simulink model "openMHA_test_db_ar_gaintable"  (R2020b)
settings: Solver=VariableStepAuto  StartTime=0.0  StopTime=stop_time  RelTol=1e-3
InitFcn:
  | initCallback
StopFcn:
  | stopCallback
values from neighbouring files (symbols this model uses):
  buf_a = 65.*ones(num_bands,1)    [test_db_ar_gaintable_init.m]
  n_ar = num_bands*2    (= 16)    [test_db_ar_gaintable_init.m]
  num_bands = 8    [test_db_ar_gaintable_init.m]
  RAM_addresses = 2^(RAM_size)    (= 256)    [test_db_ar_gaintable_init.m]
  table_length = length(gtdata)    [test_db_ar_gaintable_init.m]
  X_high = 93    [test_db_ar_gaintable_init.m]
undefined symbols (not defined in the file or in its folder): xIn
libraries: dspsrcs4 x4, FPGA_Open_Speech_Tools x4, simulink x4, hdlsllib x2
settings Model: SimulationMode=accelerator  PacingRate=200  Creator=t96f346  LastModifiedBy=tyler

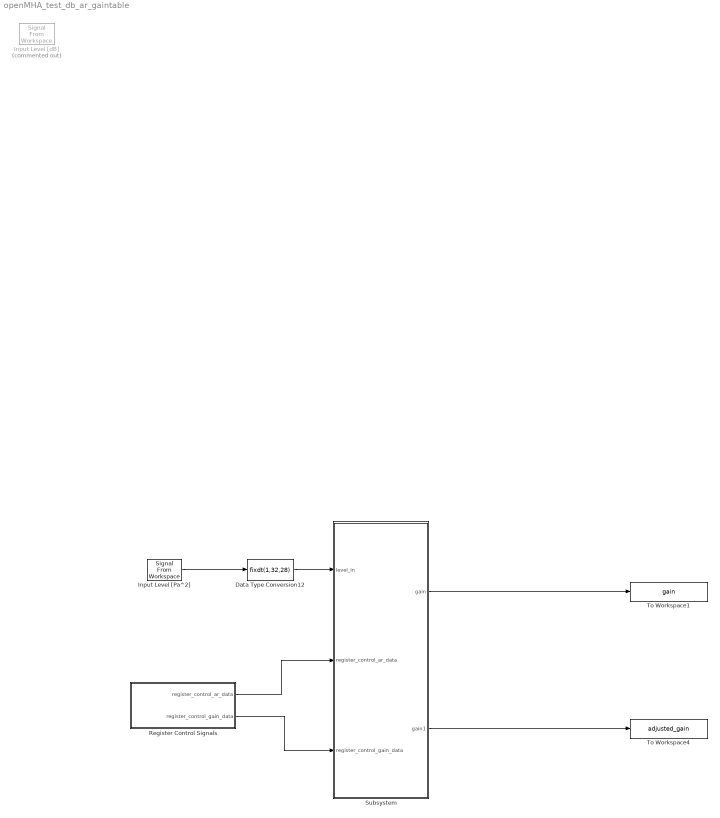
== system openMHA_test_db_ar_gaintable ==
  Data Type Conversion12 : DataTypeConversion  OutDataTypeStr=fixdt(1,32,28)
  Input Level [Pa^2] : dspsrcs4/Signal From Workspace  X=level_in  Ts=1  nsamps=1  OutputAfterFinalValue=Setting to zero  ignoreOrWarnInputAndFrameLengths=off  OutputFrames=off
  Input Level [dB] : dspsrcs4/Signal From Workspace  Commented=on  X=Lst  Ts=1  nsamps=1  OutputAfterFinalValue=Setting to zero  ignoreOrWarnInputAndFrameLengths=off  OutputFrames=off
  Register Control Signals : Subsystem
  Subsystem : Subsystem
  To Workspace1 : ToWorkspace  VariableName=gain  SampleTime=-1
      settings: Save2DSignal=2-D array (concatenate along first dimension)
  To Workspace4 : ToWorkspace  VariableName=adjusted_gain  SampleTime=-1
      settings: Save2DSignal=2-D array (concatenate along first dimension)
  wires:
  Input Level [Pa^2]/1 -> Data Type Conversion12/1
  Data Type Conversion12/1 -> Subsystem/1(level_in)
  Subsystem/1(gain) -> To Workspace1/1
  Subsystem/2(gain1) -> To Workspace4/1
  Register Control Signals/1("register_control_ar_data ") -> Subsystem/2(register_control_ar_data)
  Register Control Signals/2(register_control_gain_data) -> Subsystem/3(register_control_gain_data)

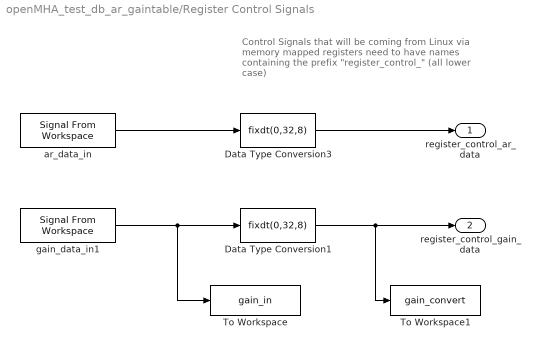
== system openMHA_test_db_ar_gaintable/Register Control Signals ==
  note: Control Signals that will be coming from Linux via
      | memory mapped registers need to have names
      | containing the prefix "register_control_"
      | (all lower case)
  Data Type Conversion1 : DataTypeConversion  OutDataTypeStr=fixdt(0,32,8)
  Data Type Conversion3 : DataTypeConversion  OutDataTypeStr=fixdt(0,32,8)
  To Workspace : ToWorkspace  VariableName=gain_in  SaveFormat=Timeseries  SampleTime=-1
  To Workspace1 : ToWorkspace  VariableName=gain_convert  SaveFormat=Timeseries  SampleTime=-1
  ar_data_in : dspsrcs4/Signal From Workspace  X=ar_data_in  Ts=1  nsamps=1  OutputAfterFinalValue=Setting to zero  ignoreOrWarnInputAndFrameLengths=off  OutputFrames=off
  gain_data_in1 : dspsrcs4/Signal From Workspace  X=gain_data_in  Ts=1  nsamps=1  OutputAfterFinalValue=Setting to zero  ignoreOrWarnInputAndFrameLengths=off  OutputFrames=off
  "register_control_ar_data " : Outport  VectorParamsAs1DForOutWhenUnconnected=off
  register_control_gain_data : Outport  Port=2  VectorParamsAs1DForOutWhenUnconnected=off
  wires:
  Data Type Conversion3/1 -> "register_control_ar_data "/1
  Data Type Conversion1/1 -> To Workspace1/1, register_control_gain_data/1
  ar_data_in/1 -> Data Type Conversion3/1
  gain_data_in1/1 -> To Workspace/1, Data Type Conversion1/1

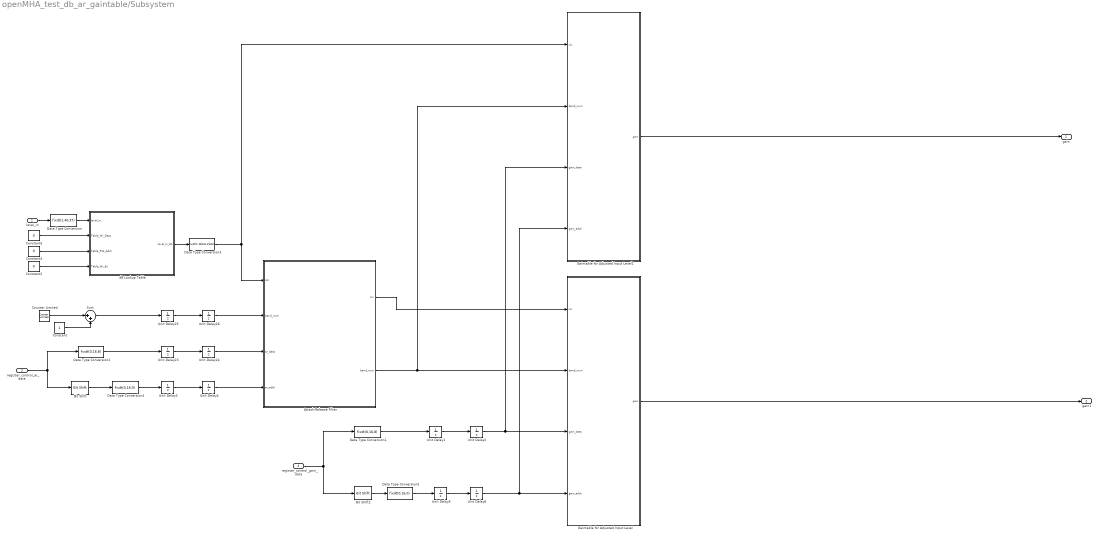
== system openMHA_test_db_ar_gaintable/Subsystem ==
  level_in : Inport
  register_control_ar_data : Inport  Port=2
  register_control_gain_data : Inport  Port=3
  Attack-Release Filter : Subsystem
  Bit Shift : hdlsllib/Logic and Bit Operations/Bit Shift  mode=Shift Right Logical  N=8
  Bit Shift1 : hdlsllib/Logic and Bit Operations/Bit Shift  mode=Shift Right Logical  N=8
  Constant : Constant
  Constant2 : Constant  Value=0  OutDataTypeStr=boolean  SampleTime=-1
  Constant4 : Constant  Value=0  OutDataTypeStr=uint16  SampleTime=-1
  Constant5 : Constant  Value=0  OutDataTypeStr=fixdt(1,40,32)  SampleTime=-1
  Counter Limited : simulink/Sources/Counter Limited  uplimit=num_bands-1  tsamp=-1
  Data Type Conversion : DataTypeConversion  OutDataTypeStr=fixdt(1,40,37)
  Data Type Conversion1 : DataTypeConversion  OutDataTypeStr=fixdt(0,16,8)
  Data Type Conversion2 : DataTypeConversion  OutDataTypeStr=fixdt(0,16,8)
  Data Type Conversion3 : DataTypeConversion  OutDataTypeStr=fixdt(1,Wbits,Fbits)
  Data Type Conversion4 : DataTypeConversion  OutDataTypeStr=fixdt(0,16,0)
  Data Type Conversion5 : DataTypeConversion  OutDataTypeStr=fixdt(0,16,0)
  Gaintable for Adjusted Input Level : Subsystem
  Gaintable for Adjusted Input Level1 : Subsystem
  Sum : Sum  Inputs=|++
  Unit Delay{1..6,23..26} (10 alike) : UnitDelay  SampleTime=-1  HasFrameUpgradeWarning=on
  dB Lookup Table : Subsystem
  gain : Outport
  gain1 : Outport  Port=2
  wires:
  Unit Delay24/1 -> Attack-Release Filter/3(ar_data)
  Data Type Conversion3/1 -> Attack-Release Filter/1(Lst), Gaintable for Adjusted Input Level1/1(Lin)
  Unit Delay26/1 -> Attack-Release Filter/2(band_num)
  Attack-Release Filter/1(Lin) -> Gaintable for Adjusted Input Level/1(Lin)
  Attack-Release Filter/2("band_num ") -> Gaintable for Adjusted Input Level1/2(band_num), Gaintable for Adjusted Input Level/2(band_num)
  Constant2/1 -> dB Lookup Table/4(Table_Wr_En)
  dB Lookup Table/1(level_in_db) -> Data Type Conversion3/1
  Data Type Conversion2/1 -> Unit Delay23/1
  Sum/1 -> Unit Delay25/1
  Unit Delay25/1 -> Unit Delay26/1
  Unit Delay23/1 -> Unit Delay24/1
  Gaintable for Adjusted Input Level1/1(gain) -> gain/1
  Constant5/1 -> dB Lookup Table/2(Table_Wr_Data)
  Gaintable for Adjusted Input Level/1(gain) -> gain1/1
  Constant4/1 -> dB Lookup Table/3(Table_RW_Addr)
  level_in/1 -> Data Type Conversion/1
  Data Type Conversion/1 -> dB Lookup Table/1(level_in)
  Counter Limited/1 -> Sum/1
  Constant/1 -> Sum/2
  register_control_ar_data/1 -> Data Type Conversion2/1, Bit Shift/1
  Unit Delay1/1 -> Unit Delay2/1
  Data Type Conversion1/1 -> Unit Delay1/1
  register_control_gain_data/1 -> Data Type Conversion1/1, Bit Shift1/1
  Unit Delay2/1 -> Gaintable for Adjusted Input Level1/3(gain_data), Gaintable for Adjusted Input Level/3(gain_data)
  Unit Delay3/1 -> Unit Delay4/1
  Unit Delay4/1 -> Attack-Release Filter/4(ar_addr)
  Unit Delay5/1 -> Unit Delay6/1
  Unit Delay6/1 -> Gaintable for Adjusted Input Level1/4(gain_addr), Gaintable for Adjusted Input Level/4(gain_addr)
  Bit Shift/1 -> Data Type Conversion4/1
  Data Type Conversion4/1 -> Unit Delay3/1
  Bit Shift1/1 -> Data Type Conversion5/1
  Data Type Conversion5/1 -> Unit Delay5/1

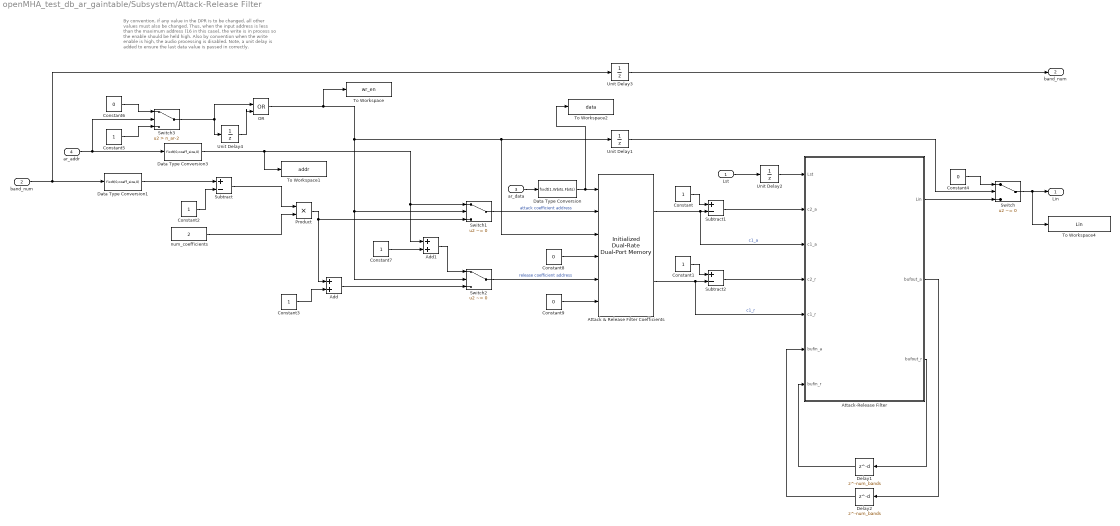
== system openMHA_test_db_ar_gaintable/Subsystem/Attack-Release Filter ==
  note: By convention, if any value in the DPR is to be changed, all other
      | values must also be changed.  Thus, when the input address is
      | less than the maximum address (16 in this case), the write is in
      | process so the enable should be held high.  Also by convention
      | when the write enable is high, the audio processing is disabled.
      | Note, a unit delay is added to ensure the last data value is passed
      | in correctly.
  Lst : Inport
  band_num : Inport  Port=2
  ar_data : Inport  Port=3
  ar_addr : Inport  Port=4
  Add : Sum
  Add1 : Sum
  Attack & Release Filter Coefficients : FPGA_Open_Speech_Tools/Initialized Dual-Rate Dual-Port Memory  ram_size=coeff_size  Table_Init=ar_coeffs
      settings: SourceProductName=FPGA Open Speech Tools
  Attack-Release Filter : Subsystem
  Constant : Constant  OutDataTypeStr=fixdt(1,Wbits,Fbits)  SampleTime=-1
  Constant1 : Constant  OutDataTypeStr=fixdt(1,Wbits,Fbits)  SampleTime=-1
  Constant2 : Constant  OutDataTypeStr=fixdt(0,coeff_size,0)  SampleTime=-1
  Constant3 : Constant  OutDataTypeStr=fixdt(0,coeff_size,0)  SampleTime=-1
  Constant4 : Constant  Value=0  OutDataTypeStr=fixdt(1,Wbits,Fbits)  SampleTime=-1
  Constant5 : Constant  OutDataTypeStr=boolean  SampleTime=-1
  Constant6 : Constant  Value=0  OutDataTypeStr=boolean  SampleTime=-1
  Constant7 : Constant  OutDataTypeStr=fixdt(0,coeff_size,0)  SampleTime=-1
  Constant8 : Constant  Value=0  OutDataTypeStr=fixdt(1,Wbits,Fbits)  SampleTime=-1
  Constant9 : Constant  Value=0  OutDataTypeStr=boolean  SampleTime=-1
  Data Type Conversion : DataTypeConversion  OutDataTypeStr=fixdt(1,Wbits,Fbits)
  Data Type Conversion1 : DataTypeConversion  OutDataTypeStr=fixdt(0,coeff_size,0)
  Data Type Conversion3 : DataTypeConversion  OutDataTypeStr=fixdt(0,coeff_size,0)
  Delay1 : Delay  DelayLength=num_bands  InitialCondition=buf_a  UseCircularBuffer=on
  Delay2 : Delay  DelayLength=num_bands  InitialCondition=buf_a  UseCircularBuffer=on
  OR : Logic  Operator=OR  IconShape=distinctive  AllPortsSameDT=off  OutDataTypeStr=boolean
  Product : Product  OutDataTypeStr=fixdt(0,coeff_size,0)
  Subtract : Sum  Inputs=+-  OutDataTypeStr=fixdt(0,coeff_size,0)
  Subtract1 : Sum  Inputs=+-  OutDataTypeStr=fixdt(1,Wbits,Fbits)
  Subtract2 : Sum  Inputs=+-  OutDataTypeStr=fixdt(1,Wbits,Fbits)
  Switch : Switch  Criteria=u2 ~= 0  OutDataTypeStr=fixdt(1,Wbits,Fbits)
  Switch1 : Switch  Criteria=u2 ~= 0  OutDataTypeStr=Inherit: Inherit via back propagation
  Switch2 : Switch  Criteria=u2 ~= 0  OutDataTypeStr=uint8
  Switch3 : Switch  Criteria=u2 > Threshold  Threshold=n_ar-2  OutDataTypeStr=boolean
  To Workspace : ToWorkspace  VariableName=wr_en  SaveFormat=Timeseries  SampleTime=-1
  To Workspace1 : ToWorkspace  VariableName=addr  SaveFormat=Timeseries  SampleTime=-1
  To Workspace2 : ToWorkspace  VariableName=data  SaveFormat=Timeseries  SampleTime=-1
  To Workspace4 : ToWorkspace  VariableName=Lin  SampleTime=-1
      settings: Save2DSignal=2-D array (concatenate along first dimension)
  Unit Delay1 : UnitDelay  SampleTime=-1  HasFrameUpgradeWarning=on
  Unit Delay2 : UnitDelay  InitialCondition=65  SampleTime=-1  HasFrameUpgradeWarning=on
  Unit Delay3 : UnitDelay  SampleTime=-1  HasFrameUpgradeWarning=on
  Unit Delay4 : UnitDelay  SampleTime=-1  HasFrameUpgradeWarning=on
  num_coefficients : Constant  Value=2  OutDataTypeStr=uint8  SampleTime=-1
  Lin : Outport
  "band_num " : Outport  Port=2
  wires:
  Delay2/1 -> Attack-Release Filter/6(bufin_a)
  Switch1/1 -> Attack & Release Filter Coefficients/2  "attack coefficient address"
  Switch2/1 -> Attack & Release Filter Coefficients/5  "release coefficient address"
  Constant8/1 -> Attack & Release Filter Coefficients/4
  Attack-Release Filter/3(bufout_r) -> Delay1/1
  Unit Delay2/1 -> Attack-Release Filter/1(Lst)
  Unit Delay1/1 -> Switch/2
  Lst/1 -> Unit Delay2/1
  Constant1/1 -> Subtract2/1
  Constant/1 -> Subtract1/1
  Switch/1 -> To Workspace4/1, Lin/1
  Attack-Release Filter/1(Lin) -> Switch/3
  Attack-Release Filter/2(bufout_a) -> Delay2/1
  OR/1 -> To Workspace/1, Unit Delay1/1, Attack & Release Filter Coefficients/3, Switch1/2, Switch2/2
  band_num/1 -> Unit Delay3/1, Data Type Conversion1/1
  Constant4/1 -> Switch/1
  Constant7/1 -> Add1/2
  Product/1 -> Switch1/3, Add/1
  Delay1/1 -> Attack-Release Filter/7(bufin_r)
  Constant3/1 -> Add/2
  Subtract2/1 -> Attack-Release Filter/4(c2_r)
  Data Type Conversion1/1 -> Subtract/1
  Subtract1/1 -> Attack-Release Filter/2(c2_a)
  Data Type Conversion3/1 -> To Workspace1/1, Add1/1, Switch1/1
  Subtract/1 -> Product/1
  num_coefficients/1 -> Product/2
  Attack & Release Filter Coefficients/2 -> Attack-Release Filter/5(c1_r), Subtract2/2  "c1_r"
  Constant2/1 -> Subtract/2
  Add/1 -> Switch2/3
  Attack & Release Filter Coefficients/1 -> Attack-Release Filter/3(c1_a), Subtract1/2  "c1_a"
  Unit Delay3/1 -> "band_num "/1
  Switch3/1 -> OR/1, Unit Delay4/1
  ar_addr/1 -> Data Type Conversion3/1, Switch3/2
  Unit Delay4/1 -> OR/2
  Constant5/1 -> Switch3/3
  Constant6/1 -> Switch3/1
  ar_data/1 -> Data Type Conversion/1
  Data Type Conversion/1 -> To Workspace2/1, Attack & Release Filter Coefficients/1
  Constant9/1 -> Attack & Release Filter Coefficients/6
  Add1/1 -> Switch2/1

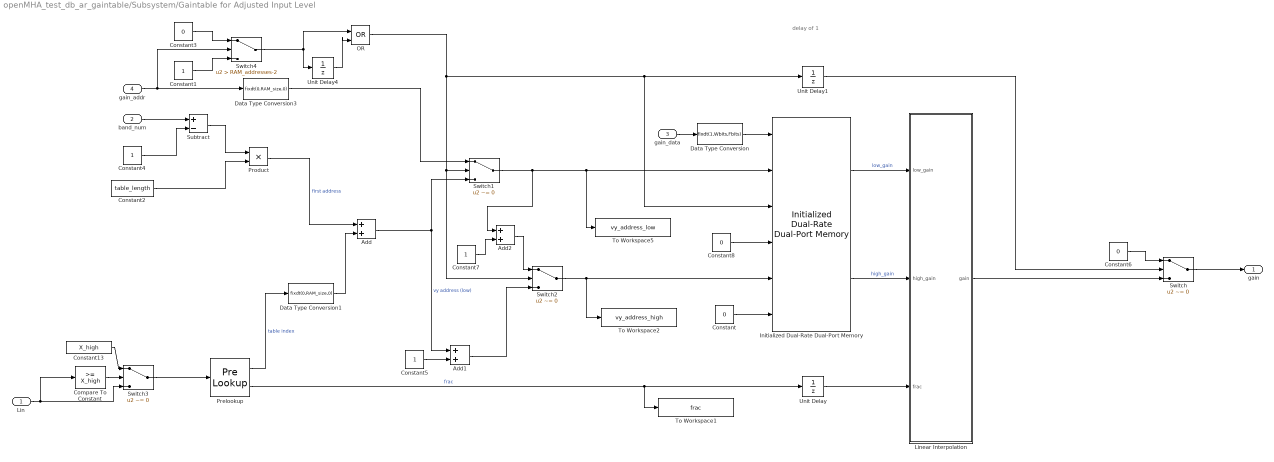
== system openMHA_test_db_ar_gaintable/Subsystem/Gaintable for Adjusted Input Level ==
  note: delay of 1
  Lin : Inport
  band_num : Inport  Port=2
  gain_data : Inport  Port=3
  gain_addr : Inport  Port=4
  Add : Sum  OutDataTypeStr=fixdt(0,RAM_size,0)
  Add1 : Sum  OutDataTypeStr=uint8
  Add2 : Sum
  Compare To Constant : simulink/Logic and Bit Operations/Compare To Constant  relop=>=  const=X_high  OutDataTypeStr=boolean
  Constant : Constant  Value=0  OutDataTypeStr=boolean  SampleTime=-1
  Constant1 : Constant  OutDataTypeStr=boolean  SampleTime=-1
  Constant13 : Constant  Value=X_high  OutDataTypeStr=fixdt(1,Wbits, Fbits)  SampleTime=-1
  Constant2 : Constant  Value=table_length  OutDataTypeStr=fixdt(0,RAM_size,0)  SampleTime=-1
  Constant3 : Constant  Value=0  OutDataTypeStr=boolean  SampleTime=-1
  Constant4 : Constant  OutDataTypeStr=fixdt(0,RAM_size,0)  SampleTime=-1
  Constant5 : Constant  OutDataTypeStr=fixdt(0,RAM_size,0)  SampleTime=-1
  Constant6 : Constant  Value=0  OutDataTypeStr=fixdt(1,16,8)  SampleTime=-1
  Constant7 : Constant  OutDataTypeStr=fixdt(0,coeff_size,0)  SampleTime=-1
  Constant8 : Constant  Value=0  OutDataTypeStr=fixdt(1,Wbits,Fbits)  SampleTime=-1
  Data Type Conversion : DataTypeConversion  OutDataTypeStr=fixdt(1,Wbits,Fbits)
  Data Type Conversion1 : DataTypeConversion  OutDataTypeStr=fixdt(0,RAM_size,0)
  Data Type Conversion3 : DataTypeConversion  OutDataTypeStr=fixdt(0,RAM_size,0)
  Initialized Dual-Rate Dual-Port Memory : FPGA_Open_Speech_Tools/Initialized Dual-Rate Dual-Port Memory  ram_size=RAM_size  Table_Init=vy
      settings: SourceProductName=FPGA Open Speech Tools
  Linear Interpolation : Subsystem
  OR : Logic  Operator=OR  IconShape=distinctive  AllPortsSameDT=off  OutDataTypeStr=boolean
  Prelookup : PreLookup  BreakpointsData=input_levels_db  IndexSearchMethod=Evenly spaced points  UseLastBreakpoint=on  DiagnosticForOutOfRangeInput=Error  IndexDataTypeStr=uint8
  Product : Product  OutDataTypeStr=Inherit: Same as first input
  Subtract : Sum  Inputs=+-
  Switch : Switch  Criteria=u2 ~= 0  OutDataTypeStr=fixdt(1,16,8)
  Switch1 : Switch  Criteria=u2 ~= 0  OutDataTypeStr=fixdt(0,RAM_size,0)
  Switch2 : Switch  Criteria=u2 ~= 0  OutDataTypeStr=fixdt(0,RAM_size,0)
  Switch3 : Switch  Criteria=u2 ~= 0
  Switch4 : Switch  Criteria=u2 > Threshold  Threshold=RAM_addresses-2  OutDataTypeStr=boolean
  To Workspace1 : ToWorkspace  VariableName=frac  SampleTime=-1
      settings: Save2DSignal=2-D array (concatenate along first dimension)
  To Workspace2 : ToWorkspace  VariableName=vy_address_high  SampleTime=-1
      settings: Save2DSignal=2-D array (concatenate along first dimension)
  To Workspace5 : ToWorkspace  VariableName=vy_address_low  SampleTime=-1
      settings: Save2DSignal=2-D array (concatenate along first dimension)
  Unit Delay : UnitDelay  SampleTime=-1  HasFrameUpgradeWarning=on
  Unit Delay1 : UnitDelay  InitialCondition=1  SampleTime=-1  HasFrameUpgradeWarning=on
  Unit Delay4 : UnitDelay  SampleTime=-1  HasFrameUpgradeWarning=on
  gain : Outport
  wires:
  Unit Delay/1 -> Linear Interpolation/3(frac)
  Unit Delay1/1 -> Switch/2
  Compare To Constant/1 -> Switch3/2
  Switch/1 -> gain/1
  band_num/1 -> Subtract/1
  Constant6/1 -> Switch/1
  Add/1 -> Switch1/3, Add1/1  "vy address (low)"
  Linear Interpolation/1(gain) -> Switch/3
  Initialized Dual-Rate Dual-Port Memory/2 -> Linear Interpolation/2(high_gain)  "high_gain"
  OR/1 -> Unit Delay1/1, Initialized Dual-Rate Dual-Port Memory/3, Switch1/2, Switch2/2
  Constant5/1 -> Add1/2
  Constant13/1 -> Switch3/1
  Add1/1 -> Switch2/3
  Initialized Dual-Rate Dual-Port Memory/1 -> Linear Interpolation/1(low_gain)  "low_gain"
  Switch2/1 -> Initialized Dual-Rate Dual-Port Memory/5, To Workspace2/1
  Constant4/1 -> Subtract/2
  Prelookup/2 -> To Workspace1/1, Unit Delay/1  "frac"
  Product/1 -> Add/1  "first address"
  Subtract/1 -> Product/1
  Lin/1 -> Compare To Constant/1, Switch3/3
  Constant2/1 -> Product/2
  Switch3/1 -> Prelookup/1
  Data Type Conversion3/1 -> Switch1/1
  Constant3/1 -> Switch4/1
  Constant1/1 -> Switch4/3
  gain_addr/1 -> Data Type Conversion3/1, Switch4/2
  Switch4/1 -> OR/1, Unit Delay4/1
  Unit Delay4/1 -> OR/2
  Add2/1 -> Switch2/1
  Constant/1 -> Initialized Dual-Rate Dual-Port Memory/6
  Constant8/1 -> Initialized Dual-Rate Dual-Port Memory/4
  gain_data/1 -> Data Type Conversion/1
  Data Type Conversion/1 -> Initialized Dual-Rate Dual-Port Memory/1
  Prelookup/1 -> Data Type Conversion1/1  "table index"
  Data Type Conversion1/1 -> Add/2
  Switch1/1 -> To Workspace5/1, Initialized Dual-Rate Dual-Port Memory/2, Add2/1
  Constant7/1 -> Add2/2

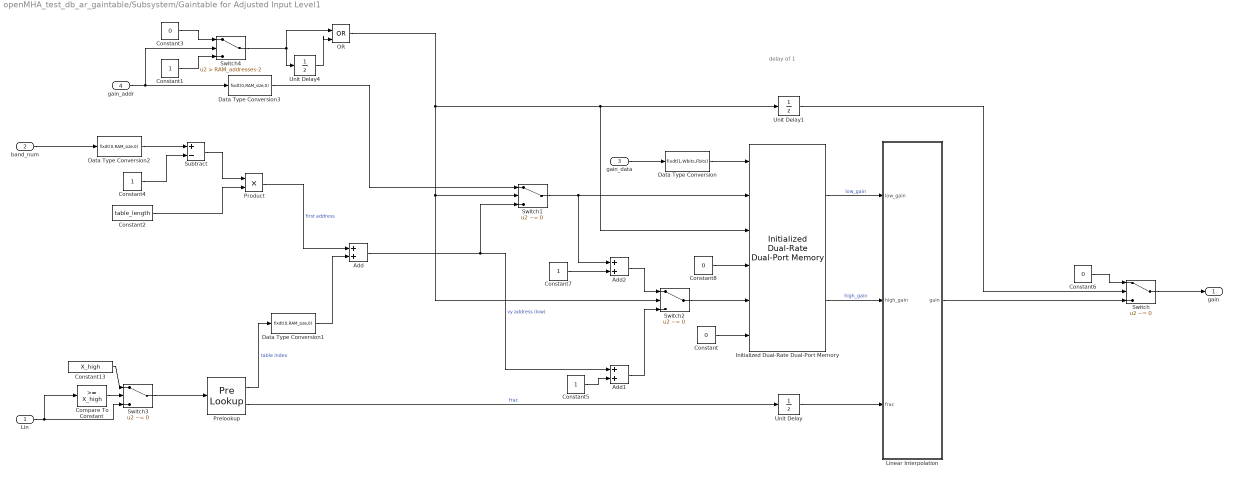
== system openMHA_test_db_ar_gaintable/Subsystem/Gaintable for Adjusted Input Level1 ==
  note: delay of 1
  Lin : Inport
  band_num : Inport  Port=2
  gain_data : Inport  Port=3
  gain_addr : Inport  Port=4
  Add : Sum  OutDataTypeStr=fixdt(0,RAM_size,0)
  Add1 : Sum  OutDataTypeStr=fixdt(0,RAM_size,0)
  Add2 : Sum
  Compare To Constant : simulink/Logic and Bit Operations/Compare To Constant  relop=>=  const=X_high  OutDataTypeStr=boolean
  Constant : Constant  Value=0  OutDataTypeStr=boolean  SampleTime=-1
  Constant1 : Constant  OutDataTypeStr=boolean  SampleTime=-1
  Constant13 : Constant  Value=X_high  OutDataTypeStr=fixdt(1,Wbits, Fbits)  SampleTime=-1
  Constant2 : Constant  Value=table_length  OutDataTypeStr=fixdt(0,RAM_size,0)  SampleTime=-1
  Constant3 : Constant  Value=0  OutDataTypeStr=boolean  SampleTime=-1
  Constant4 : Constant  OutDataTypeStr=fixdt(0,RAM_size,0)  SampleTime=-1
  Constant5 : Constant  OutDataTypeStr=fixdt(0,RAM_size,0)  SampleTime=-1
  Constant6 : Constant  Value=0  OutDataTypeStr=fixdt(1,16,8)  SampleTime=-1
  Constant7 : Constant  OutDataTypeStr=fixdt(0,coeff_size,0)  SampleTime=-1
  Constant8 : Constant  Value=0  OutDataTypeStr=fixdt(1,Wbits,Fbits)  SampleTime=-1
  Data Type Conversion : DataTypeConversion  OutDataTypeStr=fixdt(1,Wbits,Fbits)
  Data Type Conversion1 : DataTypeConversion  OutDataTypeStr=fixdt(0,RAM_size,0)
  Data Type Conversion2 : DataTypeConversion  OutDataTypeStr=fixdt(0,RAM_size,0)
  Data Type Conversion3 : DataTypeConversion  OutDataTypeStr=fixdt(0,RAM_size,0)
  Initialized Dual-Rate Dual-Port Memory : FPGA_Open_Speech_Tools/Initialized Dual-Rate Dual-Port Memory  ram_size=RAM_size  Table_Init=vy
      settings: SourceProductName=FPGA Open Speech Tools
  Linear Interpolation : Subsystem
  OR : Logic  Operator=OR  IconShape=distinctive  AllPortsSameDT=off  OutDataTypeStr=boolean
  Prelookup : PreLookup  BreakpointsData=input_levels_db  IndexSearchMethod=Evenly spaced points  UseLastBreakpoint=on  DiagnosticForOutOfRangeInput=Error  IndexDataTypeStr=uint8
  Product : Product  OutDataTypeStr=Inherit: Same as first input
  Subtract : Sum  Inputs=+-  OutDataTypeStr=fixdt(0,RAM_size,0)
  Switch : Switch  Criteria=u2 ~= 0  OutDataTypeStr=fixdt(1,16,8)
  Switch1 : Switch  Criteria=u2 ~= 0  OutDataTypeStr=fixdt(0,RAM_size,0, 'DataTypeOverride', 'Off')
  Switch2 : Switch  Criteria=u2 ~= 0  OutDataTypeStr=fixdt(0,RAM_size,0, 'DataTypeOverride', 'Off')
  Switch3 : Switch  Criteria=u2 ~= 0
  Switch4 : Switch  Criteria=u2 > Threshold  Threshold=RAM_addresses-2  OutDataTypeStr=boolean
  Unit Delay : UnitDelay  SampleTime=-1  HasFrameUpgradeWarning=on
  Unit Delay1 : UnitDelay  InitialCondition=1  SampleTime=-1  HasFrameUpgradeWarning=on
  Unit Delay4 : UnitDelay  SampleTime=-1  HasFrameUpgradeWarning=on
  gain : Outport
  wires:
  Unit Delay/1 -> Linear Interpolation/3(frac)
  Unit Delay1/1 -> Switch/2
  Compare To Constant/1 -> Switch3/2
  Switch/1 -> gain/1
  Constant6/1 -> Switch/1
  Add/1 -> Switch1/3, Add1/1  "vy address (low)"
  Linear Interpolation/1(gain) -> Switch/3
  Initialized Dual-Rate Dual-Port Memory/2 -> Linear Interpolation/2(high_gain)  "high_gain"
  OR/1 -> Unit Delay1/1, Initialized Dual-Rate Dual-Port Memory/3, Switch1/2, Switch2/2
  Constant5/1 -> Add1/2
  Constant13/1 -> Switch3/1
  Add1/1 -> Switch2/3
  Initialized Dual-Rate Dual-Port Memory/1 -> Linear Interpolation/1(low_gain)  "low_gain"
  Switch2/1 -> Initialized Dual-Rate Dual-Port Memory/5
  Constant4/1 -> Subtract/2
  Prelookup/2 -> Unit Delay/1  "frac"
  Product/1 -> Add/1  "first address"
  Subtract/1 -> Product/1
  Lin/1 -> Compare To Constant/1, Switch3/3
  Constant2/1 -> Product/2
  Switch3/1 -> Prelookup/1
  Data Type Conversion/1 -> Initialized Dual-Rate Dual-Port Memory/1
  gain_data/1 -> Data Type Conversion/1
  Unit Delay4/1 -> OR/2
  Switch4/1 -> OR/1, Unit Delay4/1
  Constant1/1 -> Switch4/3
  Constant3/1 -> Switch4/1
  gain_addr/1 -> Data Type Conversion3/1, Switch4/2
  Data Type Conversion3/1 -> Switch1/1
  Constant8/1 -> Initialized Dual-Rate Dual-Port Memory/4
  Constant/1 -> Initialized Dual-Rate Dual-Port Memory/6
  Prelookup/1 -> Data Type Conversion1/1  "table index"
  Data Type Conversion1/1 -> Add/2
  Data Type Conversion2/1 -> Subtract/1
  band_num/1 -> Data Type Conversion2/1
  Switch1/1 -> Initialized Dual-Rate Dual-Port Memory/2, Add2/1
  Constant7/1 -> Add2/2
  Add2/1 -> Switch2/1

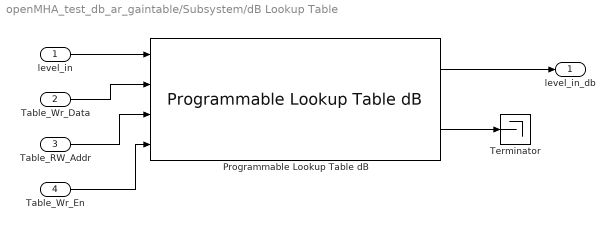
== system openMHA_test_db_ar_gaintable/Subsystem/dB Lookup Table ==
  level_in : Inport
  Table_Wr_Data : Inport  Port=2
  Table_RW_Addr : Inport  Port=3
  Table_Wr_En : Inport  Port=4
  Programmable Lookup Table dB : FPGA_Open_Speech_Tools/Programmable Lookup Table dB  tableFnParam=10.*log10(2500000000.*xIn)  SAVE_TABLE=off  maxInput=1  floorParam=2^-31  errorParam=1  ERR_DIAG=on  PLOT_TABLE=off  nBitsParam=5  mBitsParam=4  IGOTTHIS=off  W_bits=40  F_bits=37  tableInit=0  binaryOffset=0
      link override High_LUT/ram_data: InitialCondition=55.36
      link override Linear_Approximation/Unit Delay: InitialCondition=65
      link override LogAddressing/Delay1: InitialCondition=13
      link override LogAddressing/Delay2: InitialCondition=0.0001265
      link override Low_LUT/ram_data: InitialCondition=54.85
      link override Unit Delay1: InitialCondition=0.0001265
      link override Unit Delay2: InitialCondition=0.0001265
      link override Unit Delay3: InitialCondition=144
      settings: SourceProductName=FPGA Open Speech Tools
  Terminator : Terminator
  level_in_db : Outport
  wires:
  Programmable Lookup Table dB/2 -> Terminator/1
  level_in/1 -> Programmable Lookup Table dB/1
  Programmable Lookup Table dB/1 -> level_in_db/1
  Table_Wr_En/1 -> Programmable Lookup Table dB/4
  Table_Wr_Data/1 -> Programmable Lookup Table dB/2
  Table_RW_Addr/1 -> Programmable Lookup Table dB/3

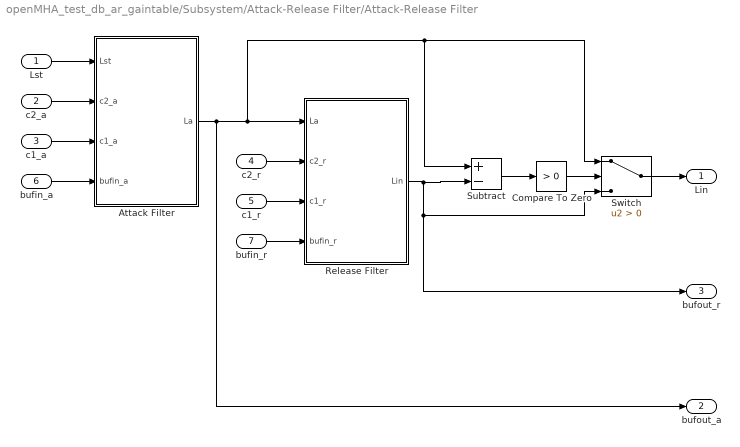
== system openMHA_test_db_ar_gaintable/Subsystem/Attack-Release Filter/Attack-Release Filter ==
  Lst : Inport
  c2_a : Inport  Port=2
  c1_a : Inport  Port=3
  c2_r : Inport  Port=4
  c1_r : Inport  Port=5
  bufin_a : Inport  Port=6
  bufin_r : Inport  Port=7
  Attack Filter : Subsystem  TreatAsAtomicUnit=on
  Compare To Zero : simulink/Logic and Bit Operations/Compare To Zero  relop=>  OutDataTypeStr=boolean
  Release Filter : Subsystem  TreatAsAtomicUnit=on
  Subtract : Sum  Inputs=+-  OutDataTypeStr=fixdt(0,Wbits,Fbits)
  Switch : Switch  Criteria=u2 > Threshold  OutDataTypeStr=fixdt(0,Wbits,Fbits)
  Lin : Outport  VectorParamsAs1DForOutWhenUnconnected=off
  bufout_a : Outport  Port=2  VectorParamsAs1DForOutWhenUnconnected=off
  bufout_r : Outport  Port=3  VectorParamsAs1DForOutWhenUnconnected=off
  wires:
  Lst/1 -> Attack Filter/1(Lst)
  c2_a/1 -> Attack Filter/2(c2_a)
  c1_a/1 -> Attack Filter/3(c1_a)
  bufin_a/1 -> Attack Filter/4(bufin_a)
  c2_r/1 -> Release Filter/2(c2_r)
  c1_r/1 -> Release Filter/3(c1_r)
  bufin_r/1 -> Release Filter/4(bufin_r)
  Attack Filter/1(La) -> bufout_a/1, Switch/1, Subtract/1, Release Filter/1(La)
  Compare To Zero/1 -> Switch/2
  Release Filter/1(Lin) -> Subtract/2, Switch/3, bufout_r/1
  Subtract/1 -> Compare To Zero/1
  Switch/1 -> Lin/1

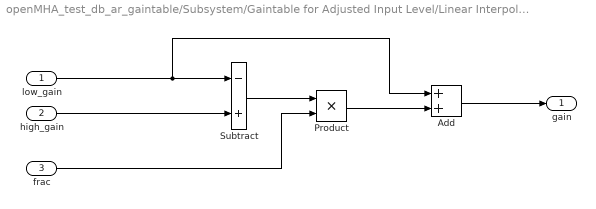
== system openMHA_test_db_ar_gaintable/Subsystem/Gaintable for Adjusted Input Level/Linear Interpolation ==
  low_gain : Inport
  high_gain : Inport  Port=2
  frac : Inport  Port=3
  Add : Sum
  Product : Product  OutDataTypeStr=Inherit: Same as first input
  Subtract : Sum  Inputs=-+
  gain : Outport
  wires:
  high_gain/1 -> Subtract/2
  low_gain/1 -> Add/1, Subtract/1
  Subtract/1 -> Product/1
  frac/1 -> Product/2
  Product/1 -> Add/2
  Add/1 -> gain/1

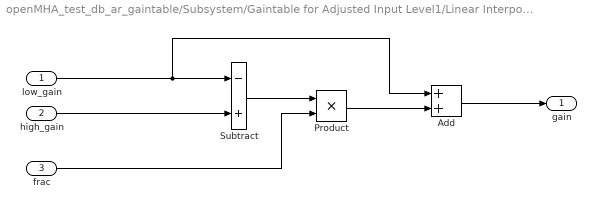
== system openMHA_test_db_ar_gaintable/Subsystem/Gaintable for Adjusted Input Level1/Linear Interpolation ==
  low_gain : Inport
  high_gain : Inport  Port=2
  frac : Inport  Port=3
  Add : Sum
  Product : Product  OutDataTypeStr=Inherit: Same as first input
  Subtract : Sum  Inputs=-+
  gain : Outport
  wires:
  high_gain/1 -> Subtract/2
  low_gain/1 -> Add/1, Subtract/1
  Subtract/1 -> Product/1
  frac/1 -> Product/2
  Product/1 -> Add/2
  Add/1 -> gain/1

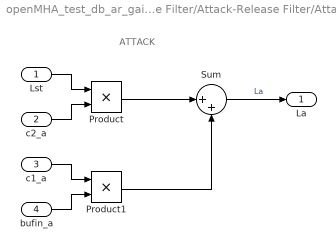
== system openMHA_test_db_ar_gaintable/Subsystem/Attack-Release Filter/Attack-Release Filter/Attack Filter ==
  note: ATTACK
  Lst : Inport
  c2_a : Inport  Port=2
  c1_a : Inport  Port=3
  bufin_a : Inport  Port=4
  Product : Product  OutDataTypeStr=fixdt(0,Wbits,Fbits)
  Product1 : Product  OutDataTypeStr=fixdt(0,Wbits,Fbits)
  Sum : Sum  Inputs=|++  OutDataTypeStr=fixdt(0,Wbits,Fbits)
  La : Outport  InitialOutput=0  VectorParamsAs1DForOutWhenUnconnected=off
  wires:
  Lst/1 -> Product/1
  Product/1 -> Sum/1
  Sum/1 -> La/1  "La"
  bufin_a/1 -> Product1/2
  Product1/1 -> Sum/2
  c2_a/1 -> Product/2
  c1_a/1 -> Product1/1

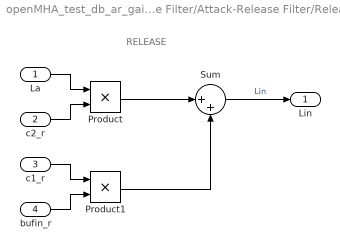
== system openMHA_test_db_ar_gaintable/Subsystem/Attack-Release Filter/Attack-Release Filter/Release Filter ==
  note: RELEASE
  La : Inport
  c2_r : Inport  Port=2
  c1_r : Inport  Port=3
  bufin_r : Inport  Port=4
  Product : Product  OutDataTypeStr=fixdt(0,Wbits,Fbits)
  Product1 : Product  OutDataTypeStr=fixdt(0,Wbits,Fbits)
  Sum : Sum  Inputs=|++  OutDataTypeStr=fixdt(0,Wbits,Fbits)
  Lin : Outport  InitialOutput=0  VectorParamsAs1DForOutWhenUnconnected=off
  wires:
  Sum/1 -> Lin/1  "Lin"
  c2_r/1 -> Product/2
  c1_r/1 -> Product1/1
  La/1 -> Product/1
  Product1/1 -> Sum/2
  Product/1 -> Sum/1
  bufin_r/1 -> Product1/2
